simulink model "Practica6_Simulink"  (R2024a)
settings: Solver=VariableStepAuto  StartTime=0.0  StopTime=0.01  RelTol=1e-3
settings Model: Creator=52331  LastModifiedBy=52331

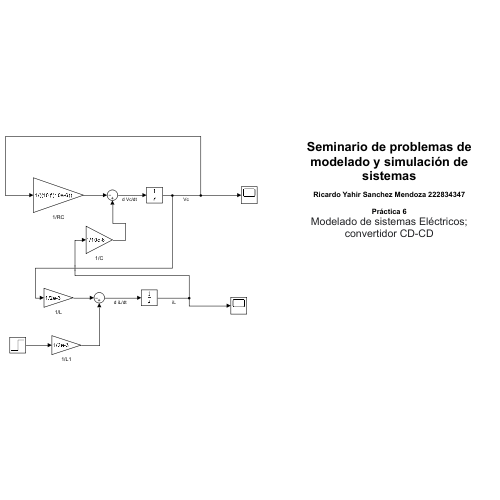
[thumbnail: Simulink's stored preview of the top-level diagram]
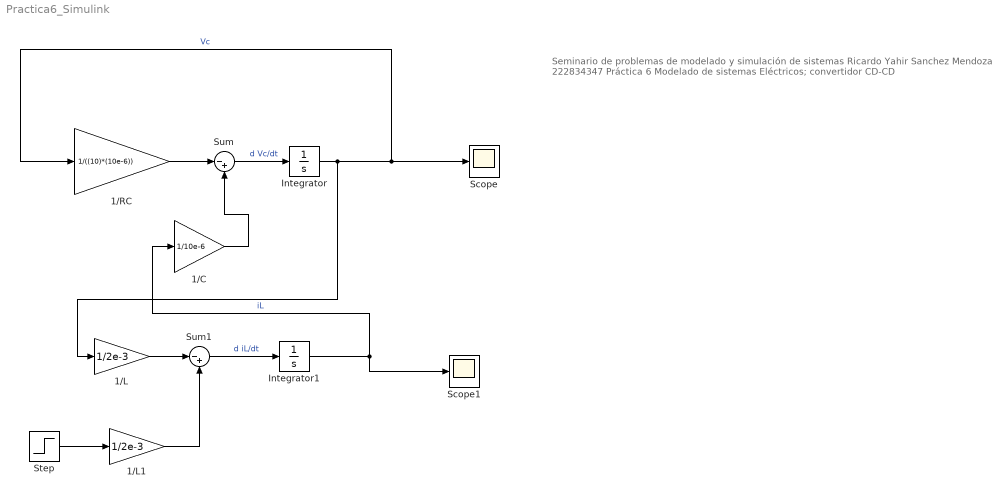
== system Practica6_Simulink ==
  note: Seminario de problemas de modelado y simulación de sistemas
      |
      | Ricardo Yahir Sanchez Mendoza 222834347
      |
      | Práctica 6
      | Modelado de sistemas Eléctricos; convertidor CD-CD
  1/C : Gain  Gain=1/10e-6
  1/L : Gain  Gain=1/2e-3
  1/L1 : Gain  Gain=1/2e-3
  1/RC : Gain  Gain=1/((10)*(10e-6))
  Integrator : Integrator
  Integrator1 : Integrator
  Scope : Scope
  Scope1 : Scope
  Step : Step  Time=0  After=32  SampleTime=0
  Sum : Sum  Inputs=|-+
  Sum1 : Sum  Inputs=|-+
  wires:
  Integrator1/1 -> 1/C/1, Scope1/1  "iL"
  Integrator/1 -> 1/L/1, Scope/1, 1/RC/1  "Vc"
  1/C/1 -> Sum/2
  1/RC/1 -> Sum/1
  Sum/1 -> Integrator/1  "d Vc/dt"
  1/L/1 -> Sum1/1
  Step/1 -> 1/L1/1
  1/L1/1 -> Sum1/2
  Sum1/1 -> Integrator1/1  "d iL/dt"
